simulink model "uz_endat_interface_2025b"  (R2025b)
settings: Solver=FixedStepDiscrete  StartTime=0.0  StopTime=1.3e-3  RelTol=1e-3
values from neighbouring files (symbols this model uses):
  binary_or_gray = false    [uz_endat_interface_init.m]
  bit_sum = endat_encoder_bit_width_multi_turn+endat_encoder_bit_width_single_turn+endat_encoder_number_of_CRC_bits    [uz_endat_interface_init.m]
  delay_first_clk_on_off = true    [uz_endat_interface_init.m]
  endat_clk_divider = 25    [uz_endat_interface_init.m]
  endat_encoder_bit_width_multi_turn = uint32(12)    [uz_endat_interface_init.m]
  endat_encoder_bit_width_single_turn = uint32(25)    [uz_endat_interface_init.m]
  endat_encoder_number_of_CRC_bits = uint32(0)    [uz_endat_interface_init.m]
  f_ADC = 20e3    (= 20000)    [uz_endat_interface_init.m]
  f_clock = 100e6    (= 100000000)    [uz_endat_interface_init.m]
  t_ADC = 1/f_ADC    (= 5e-05)    [uz_endat_interface_init.m]
  t_clock = 1/f_clock    (= 1e-08)    [uz_endat_interface_init.m]
undefined symbols (not defined in the file or in its folder): PLL
libraries: simulink x37, hdlsllib x32, simulink_extras x14, spsSampleandHoldLib x1
(part 3 of 3)

== matlab function uz_endat_interface_2025b/endat_encoder_Heidenhain_MT12bit_ST25bit/create_ST_and_MT_position_values/calc_crc ==
  data: clocks input; crc output; error1 input; error2 input; endat22 input; highpos input; lowpos input
function crc = MakeCrcPos(clocks, error1, error2, endat22, highpos, lowpos)
    % Initialize Flip-Flops
    ff = ones(1,5);  % 5 flip-flops set to 1
    code = zeros(1,66); % data bit array
    
    % Load alarm bits into code array
    if endat22
        code(1) = error1;
        code(2) = error2;
        startIdx = 1;
    else
        code(2) = error1;
        startIdx = 2;
    end
    
    % Load lowpos bits into code array
    for i = 3:34
        code(i) = bitand(lowpos, 1);
        lowpos = bitshift(lowpos, -1);
    end
    
    % Load highpos bits into code array
    for i = 35:66
        code(i) = bitand(highpos, 1);
        highpos = bitshift(highpos, -1);
    end
    
    % CRC calculation
    for i = startIdx:(clocks+2)  % adjust because MATLAB 1-based
        ex = xor(ff(5), code(i));
        ff_new = ff;
        ff_new(5) = ff(4);
        ff_new(4) = xor(ff(3), ex);
        ff_new(3) = ff(2);
        ff_new(2) = xor(ff(1), ex);
        ff_new(1) = ex;
        ff = ff_new;
    end
    
    % Store CRC in variable
    crc_tmp = 0;
    for i = 5:-1:1
        bitVal = ~ff(i);
        crc_tmp = bitshift(crc_tmp,1);
        crc_tmp = bitor(crc_tmp, bitVal);
    end
    crc=crc_tmp;
end

== matlab function uz_endat_interface_2025b/endat_encoder_Heidenhain_MT12bit_ST25bit/MATLAB Function4 ==
  data: u input; y output; cnt input
function y = fcn(u,cnt)
%#codegen
tmp = bitget(u,cnt+1);
y = tmp;

== matlab function uz_endat_interface_2025b/endat_encoder_Heidenhain_MT12bit_ST25bit/create_ST_and_MT_position_values/MATLAB Function3 ==
  data: u input; y output
function y = reverseBits(u)
%#codegen
% Reverse bit order for an unsigned fixed-point input (ufixN)

    % Determine word length from type
    BW = numerictype(u).WordLength;

    % Prepare output with same numerictype
    y = fi(0, numerictype(u), fimath(u));

    tmp = u;

    % Bit-by-bit reversal
    for i = 0:(BW-1)
        % Extract LSB, shift to MSB side, OR accumulate
        y = bitor(y, bitshift(bitand(tmp, fi(1, numerictype(u))), BW-1-i));
        tmp = bitshift(tmp, -1);
    end
end

== matlab function uz_endat_interface_2025b/uz_endat_interface/serial_communication/MATLAB Function1 ==
  data: clocks input; crc output; error1 input; error2 input; endat22 input; highpos input; lowpos input
function crc = MakeCrcPos(clocks, error1, error2, endat22, highpos, lowpos)
    % Initialize Flip-Flops
    ff = fi(ones(1,5),0,5,0);  % 5 flip-flops set to 1
    code = fi(zeros(1,64),0,64,0); % data bit array
    i = int32(0);

    
    % Load alarm bits into code array
    % if endat22
    %     code(1) = error1;
    %     code(2) = error2;
    %     startIdx = int32(1);
    % else
    %     code(2) = error1;
    %     startIdx = int32(2);
    % end
    
    % Load lowpos bits into code array
    for i = int32(3):int32(34)
        code(i) = bitand(lowpos, 1);
        lowpos = bitshift(lowpos, -1);
    end
    
    % Load highpos bits into code array
    for i = int32(35):int32(64)
        code(i) = bitand(highpos, 1);
        highpos = bitshift(highpos, -1);
    end
    
    % CRC calculation
    for i = int32(2):(int32(37)+int32(2))  % adjust because MATLAB 1-based
    % for i = startIdx:(clocks+int32(2))  % adjust because MATLAB 1-based
        ex = xor(ff(5), code(i));
        ff_new = ff;
        ff_new(5) = ff(4);
        ff_new(4) = xor(ff(3), ex);
        ff_new(3) = ff(2);
        ff_new(2) = xor(ff(1), ex);
        ff_new(1) = ex;
        ff = fi(ff_new,0,5,0);
    end
    
    % Store CRC in variable
    crc = uint32(0);
    for i = int32(5):int32(-1):int32(1)
        bitVal = uint32(~ff(i));
        crc = bitshift(crc,1);
        crc = bitor(crc, bitVal);
    end
end
